simulink model "TEST_TCP"  (R2022b)
settings: Solver=FixedStepAuto  StartTime=0.0  StopTime=inf  FixedStep=1e-3  RelTol=1e-3  EnableMultiTasking=on
undefined symbols (not defined in the file or in its folder): angular, CIRCUIT, CLTF_DAMP, CLTF_FREQ, CLTF_GAIN, CONTROL, CONTROL_INI, DiscIntNeverNeededParam, INPUT, linear, MCP3201, MD25, MODEL, MODEL_INI, mpcstate, MPU60X0, MPU9250, MSG, NAV_MPC_CONTROL, OUTPUT, RCRX, SAMPLING_TIME, SYSID_INPUT, VL6180X
libraries: raspberrypiCommlib x156, simulink x86, dspsigattribs x14, raspberrypiNetworklib x13, embedlinuxBasiclib x9, ctrlSharedLib x2, ros2lib x2, mpclib x1, vrlib x1, sldrtlib x1
(part 15 of 17)

== matlab function TEST_TCP/HARDWARE/COMMUNICATIONS/TCP//IP RPI4/RPI4 DECODER ==
  data: CONTROL_IN input; RX_MSG input; CONTROL output Bus: CONTROL_Bus; STATUS input
function CONTROL  = RPI4_DECODER(CONTROL_IN,RX_MSG,STATUS)
% Initialization
CONTROL = CONTROL_IN;
%%%%%%%%%%%%%%%%%%%%%%%%%%%%%%%%%%%%%%%%%%%%%%%%%%%%%%%%%%%%%%%%%%%%%%%%%%%
% MCS MESSAGES
%%%%%%%%%%%%%%%%%%%%%%%%%%%%%%%%%%%%%%%%%%%%%%%%%%%%%%%%%%%%%%%%%%%%%%%%%%%
% RPi4 --> RPi3 (decoder)
%       Referencia velocidad (24B): 3 single (float32) XYZ y 3 single RPY
%       Referencia pose (24B): 3 single posición XYZ y 3 single orientación XYZ
%       Pose real (24B): 3 single posición XYZ y 3 single orientación XYZ
%       GPS (24B): 3 double (float64) latitud, longitud, altitud
%       Botones (3B): 3 bool (uint8) A, B, C
%       Estado (1B): 1 byte (uint8)
%       Corriente de carga (4B): 1 single (float32)
%       Puntos lidar (960B): 120 single [distancia, ángulo]
%       TOTAL: 1064B
% WRITE IN THE CONTROL BUS
if STATUS==1
    ii = 4; jj = 4;
    CONTROL.TARGET.FORWARD_VEL_REF = double(typecast(RX_MSG(ii-jj+1:ii),'single'));
    ii = 6*4; 
    CONTROL.TARGET.YAW_RATE_REF = double(typecast(RX_MSG(ii-jj+1:ii),'single'));
    ii = 7*4;
    CONTROL.TARGET.NAV_REF_PC(1) = double(typecast(RX_MSG(ii-jj+1:ii),'single'));
    ii = 8*4;
    CONTROL.TARGET.NAV_REF_PC(2) = double(typecast(RX_MSG(ii-jj+1:ii),'single'));
    ii = 12*4;
    CONTROL.TARGET.YAW_ANG_REF = double(typecast(RX_MSG(ii-jj+1:ii),'single'));
    if CONTROL.STATE.NAV_MODE>2
        ii = 13*4;
        CONTROL.INPUT.NAV_EARTH_POS(1) = double(typecast(RX_MSG(ii-jj+1:ii),'single'));
        ii = 14*4;
        CONTROL.INPUT.NAV_EARTH_POS(2) = double(typecast(RX_MSG(ii-jj+1:ii),'single'));
    end
    ii = 18*4;
    CONTROL.INPUT.YAW_ANG = double(typecast(RX_MSG(ii-jj+1:ii),'single'));
    ii = 18*4 + 3*8 + 1; jj = 1;
    CONTROL.STATE.PC_BUTTONS(1) = RX_MSG(ii-jj+1:ii);
    ii = 18*4 + 3*8 + 2;
    CONTROL.STATE.PC_BUTTONS(2) = RX_MSG(ii-jj+1:ii);
    ii = 18*4 + 3*8 + 3; 
    CONTROL.STATE.PC_BUTTONS(3) = RX_MSG(ii-jj+1:ii);
    ii = 18*4 + 3*8 + 4;
    % CONTROL.STATE.CURRENT_STATUS_RPI4 = RX_MSG(ii-jj+1:ii);
    unused_local_variable = RX_MSG(ii-jj+1:ii);
    ii = 19*4 + 3*8 + 4; jj = 4;
    CONTROL.INPUT.CHARGING_CURRENT = double(typecast(RX_MSG(ii-jj+1:ii),'single'));
    for nn = 1:120
        CONTROL.INPUT.LIDAR_2D(nn,1) = double(typecast(RX_MSG(ii+8*nn-4:-1:ii+8*(nn-1)+1),'single'));
        CONTROL.INPUT.LIDAR_2D(nn,2) = double(typecast(RX_MSG(ii+8*nn:-1:ii+8*nn-3),'single'));
    end
end
%%%%%%%%%%%%%%%%%%%%%%%%%%%%%%%%%%%%%%%%%%%%%%%%%%%%%%%%%%%%%%%%%%%%%%%%%%%


return
